simulink model "SF011A_EotLrng"  (R2013b)
settings: Solver=FixedStepDiscrete  SolverMode=SingleTasking  StartTime=0.0  StopTime=1  FixedStep=0.002  RelTol=1e-3
values from neighbouring files (symbols this model uses):
  ARCHGLBPRM_FLOATZEROTHD_ULS_F32 = DataDict.Constant    [SF011A_EotLrng_DataDict.m]
  CNVTOMILLISEC_MILLISECPERCNT_F32 = DataDict.Constant    [SF011A_EotLrng_DataDict.m]
  CORRLNFLT_CNT_U08 = DataDict.Constant    [SF011A_EotLrng_DataDict.m]
  DEBSTEP_CNT_U16 = DataDict.Constant    [SF011A_EotLrng_DataDict.m]
  EOTLIMDETD_CNT_LOGL = DataDict.Constant    [SF011A_EotLrng_DataDict.m]
  EOTLIMNOTDETD_CNT_LOGL = DataDict.Constant    [SF011A_EotLrng_DataDict.m]
  EotLrngAuthyStrtLrn = DataDict.Calibration    [SF011A_EotLrng_DataDict.m]
  EotLrngEotLrnTmr = DataDict.Calibration    [SF011A_EotLrng_DataDict.m]
  EotLrngHwAgOverTrvlCnt = DataDict.Calibration    [SF011A_EotLrng_DataDict.m]
  EotLrngHwAgOverTrvlEntr = DataDict.Calibration    [SF011A_EotLrng_DataDict.m]
  EotLrngHwAgOverTrvlExit = DataDict.Calibration    [SF011A_EotLrng_DataDict.m]
  EotLrngHwTqEotLrn = DataDict.Calibration    [SF011A_EotLrng_DataDict.m]
  EotLrngMotVelEotLrn = DataDict.Calibration    [SF011A_EotLrng_DataDict.m]
  EotLrngRackTrvlMax = DataDict.Calibration    [SF011A_EotLrng_DataDict.m]
  EotLrngRackTrvlMin = DataDict.Calibration    [SF011A_EotLrng_DataDict.m]
  EotLrngRstAuthyMin = DataDict.Calibration    [SF011A_EotLrng_DataDict.m]
  EotProtnRackTrvlLimrEna = DataDict.ImprtdCal    [SF011A_EotLrng_DataDict.m]
  HwAgOverTrvl = DataDict.NTC    [SF011A_EotLrng_DataDict.m]
  HWAGOVERTRVLMAXCNT_CNT_U08 = DataDict.Constant    [SF011A_EotLrng_DataDict.m]
  NODEBSTEP_CNT_U16 = DataDict.Constant    [SF011A_EotLrng_DataDict.m]
  OUTOFRNGFLT_CNT_U08 = DataDict.Constant    [SF011A_EotLrng_DataDict.m]
  RackEotStorgFlt = DataDict.NTC    [SF011A_EotLrng_DataDict.m]
  SIGAVLFLT_CNT_U08 = DataDict.Constant    [SF011A_EotLrng_DataDict.m]
undefined symbols (not defined in the file or in its folder): NtcSts1, NvmGetErrSts1, SigQlfr1
libraries: simulink x19, NxtrNvM x12, NxtrAbslt x5, NxtrLim x4, NxtrMax x3, NxtrMin x3
(part 4 of 7)

== system SF011A_EotLrng/EotLrng/EotLrngPer1/SRLNotEna/CalcResetEot ==
  HwAgDiDiagSts : Inport  RequirementInfo="{'linktype_rmi_doors' '0000ba59 (/E-STEER Core/SubSystem Specifications/Application Functions/SF011A Learned EOT Limits)' '#SF011A_79' 'true' 'REQ:  SF011A_79' '' } %GIDa_e08988e2_1562_4c51_b269_de6339d57bf1"
  HwAuthy : Inport  RequirementInfo="{'linktype_rmi_doors' '0000ba59 (/E-STEER Core/SubSystem Specifications/Application Functions/SF011A Learned EOT Limits)' '#SF011A_80' 'true' 'REQ:  SF011A_80' '' ; 'linktype_rmi_doors' '0000ba59 (/E-STEER Core/SubSystem Specifications/Application Functions/SF011A Learned EOT Limits)' '#SF011A_81' 'true' 'REQ:  SF011A_81' '' } %GIDa_5c7a69a0_a64f_4965_bcc2_68fe0bcf48ea"  Port=2
  HwAg : Inport  Port=3
  Calibration : Constant  RequirementInfo="{'linktype_rmi_doors' '0000ba59 (/E-STEER Core/SubSystem Specifications/Application Functions/SF011A Learned EOT Limits)' '#SF011A_80' 'true' 'REQ:  SF011A_80' '' ; 'linktype_rmi_doors' '0000ba59 (/E-STEER Core/SubSystem Specifications/Application Functions/SF011A Learned EOT Limits)' '#SF011A_81' 'true' 'REQ:  SF011A_81' '' } %GIDa_1b637f2f_e852_4a1f_a59d_2b9db53c6dd7"  Value=EotLrngRstAuthyMin
  Constant3 : Constant  RequirementInfo="{'linktype_rmi_doors' '0000ba59 (/E-STEER Core/SubSystem Specifications/Application Functions/SF011A Learned EOT Limits)' '#SF011A_80' 'true' 'REQ:  SF011A_80' '' ; 'linktype_rmi_doors' '0000ba59 (/E-STEER Core/SubSystem Specifications/Application Functions/SF011A Learned EOT Limits)' '#SF011A_81' 'true' 'REQ:  SF011A_81' '' } %GIDa_fd907c25_ae57_48e9_8be4_a6bebbc957dd"  Value=EotLrngRackTrvlMax
  Constant4 : Constant  RequirementInfo="{'linktype_rmi_doors' '0000ba59 (/E-STEER Core/SubSystem Specifications/Application Functions/SF011A Learned EOT Limits)' '#SF011A_81' 'true' 'REQ:  SF011A_81' '' ; 'linktype_rmi_doors' '0000ba59 (/E-STEER Core/SubSystem Specifications/Application Functions/SF011A Learned EOT Limits)' '#SF011A_80' 'true' 'REQ:  SF011A_80' '' } %GIDa_3d9f2888_eef3_40f6_8ef6_142645e82430"  Value=EotLrngRackTrvlMax
  CopyRight2 : Subsystem  Description=|  mask(Copyright Information){none=on}
      | Copyright info block.                                               
      |                                                                     
      | Place copyright information at the top of every subsystem in design.
      mask prompts: none "No parameters"
      mask help: Place copyright information at the top of every subsystem in design.
      mask Display:
      | NxtrConf = 'Nexteer Confidential';
      | 
      | sys = bdroot; %handle for the current model ("system")
      | first = get_param(sys,'Created');
      | if(isempty(first))
      |     first = datestr(now,'yyyy');
      | else
      |     first = first(end-3:end);  %year is last four digits
      | end
      | 
      | last = get_param(sys,'LastModifiedDate');
      | if isempty(last)
      |     last = datestr(now,'yyyy');
      | else
      |     last = last(end-3:end);
      | end
      | 
      | if strcmp(first,last)
      |     fprintf('%s -- Copyright %s Nexteer',NxtrConf,first)
      | else
      |     fprintf('%s -- %s%s- %s Nexteer',NxtrConf,char(169),first,last)
      | end
  Data Store Read1 : DataStoreRead  RequirementInfo="{'linktype_rmi_doors' '0000ba59 (/E-STEER Core/SubSystem Specifications/Application Functions/SF011A Learned EOT Limits)' '#SF011A_78' 'true' 'REQ:  SF011A_78' '' } %GIDa_dc92841a_08af_4fc8_a8e8_ed04e745d80a"  DataStoreName=RstLimReq
  Logical Operator : Logic  RequirementInfo="{'linktype_rmi_doors' '0000ba59 (/E-STEER Core/SubSystem Specifications/Application Functions/SF011A Learned EOT Limits)' '#SF011A_78' 'true' 'REQ:  SF011A_78' '' ; 'linktype_rmi_doors' '0000ba59 (/E-STEER Core/SubSystem Specifications/Application Functions/SF011A Learned EOT Limits)' '#SF011A_79' 'true' 'REQ:  SF011A_79' '' ; 'linktype_rmi_doors' '0000ba59 (/E-STEER Core/SubSystem Specifications/Application Functions/SF011A Learned EOT Limits)' '#SF011A_80' 'true' 'REQ:  SF011A_80' '' ; 'linktype_rmi_doors' '0000ba59 (/E-STEER Core/SubSystem Specifications/Application Functions/SF011A Learned EOT Limits)' '#SF011A_81' 'true' 'REQ:  SF011A_81' '' } %GIDa_11ff6ad1_50e6_4918_a9aa_75679ebe76f8"  Operator=OR  Inputs=3  AllPortsSameDT=off  OutDataTypeStr=boolean
  Logical Operator1 : Logic  RequirementInfo="{'linktype_rmi_doors' '0000ba59 (/E-STEER Core/SubSystem Specifications/Application Functions/SF011A Learned EOT Limits)' '#SF011A_80' 'true' 'REQ:  SF011A_80' '' ; 'linktype_rmi_doors' '0000ba59 (/E-STEER Core/SubSystem Specifications/Application Functions/SF011A Learned EOT Limits)' '#SF011A_81' 'true' 'REQ:  SF011A_81' '' } %GIDa_2555febd_936c_40b2_9f9b_c08210222f29"  Operator=OR  AllPortsSameDT=off  OutDataTypeStr=boolean
  Logical Operator2 : Logic  RequirementInfo="{'linktype_rmi_doors' '0000ba59 (/E-STEER Core/SubSystem Specifications/Application Functions/SF011A Learned EOT Limits)' '#SF011A_80' 'true' 'REQ:  SF011A_80' '' ; 'linktype_rmi_doors' '0000ba59 (/E-STEER Core/SubSystem Specifications/Application Functions/SF011A Learned EOT Limits)' '#SF011A_81' 'true' 'REQ:  SF011A_81' '' } %GIDa_6e14db6e_5a83_4e69_9a75_17202af61501"  AllPortsSameDT=off  OutDataTypeStr=boolean
  Relational Operator : RelationalOperator  RequirementInfo="{'linktype_rmi_doors' '0000ba59 (/E-STEER Core/SubSystem Specifications/Application Functions/SF011A Learned EOT Limits)' '#SF011A_80' 'true' 'REQ:  SF011A_80' '' ; 'linktype_rmi_doors' '0000ba59 (/E-STEER Core/SubSystem Specifications/Application Functions/SF011A Learned EOT Limits)' '#SF011A_81' 'true' 'REQ:  SF011A_81' '' } %GIDa_a3ca0082_78b3_49a3_89f7_5ece7a959c8e"  OutDataTypeStr=boolean
  Relational Operator2 : RelationalOperator  RequirementInfo="{'linktype_rmi_doors' '0000ba59 (/E-STEER Core/SubSystem Specifications/Application Functions/SF011A Learned EOT Limits)' '#SF011A_80' 'true' 'REQ:  SF011A_80' '' ; 'linktype_rmi_doors' '0000ba59 (/E-STEER Core/SubSystem Specifications/Application Functions/SF011A Learned EOT Limits)' '#SF011A_81' 'true' 'REQ:  SF011A_81' '' } %GIDa_389cdd7e_2d79_4d3e_a6fc_d51a3a0d06bf"  Operator=>  OutDataTypeStr=boolean
  Relational Operator3 : RelationalOperator  RequirementInfo="{'linktype_rmi_doors' '0000ba59 (/E-STEER Core/SubSystem Specifications/Application Functions/SF011A Learned EOT Limits)' '#SF011A_81' 'true' 'REQ:  SF011A_81' '' ; 'linktype_rmi_doors' '0000ba59 (/E-STEER Core/SubSystem Specifications/Application Functions/SF011A Learned EOT Limits)' '#SF011A_80' 'true' 'REQ:  SF011A_80' '' } %GIDa_7abd7096_ec6f_448b_88cf_8cd7c03d0901"  Operator=<  OutDataTypeStr=boolean
  Unary Minus : UnaryMinus  RequirementInfo="{'linktype_rmi_doors' '0000ba59 (/E-STEER Core/SubSystem Specifications/Application Functions/SF011A Learned EOT Limits)' '#SF011A_81' 'true' 'REQ:  SF011A_81' '' ; 'linktype_rmi_doors' '0000ba59 (/E-STEER Core/SubSystem Specifications/Application Functions/SF011A Learned EOT Limits)' '#SF011A_80' 'true' 'REQ:  SF011A_80' '' } %GIDa_d6db76b3_3df1_4d39_8e0a_09f1875fa956"
  RstEot : Outport  RequirementInfo="{'linktype_rmi_doors' '0000ba59 (/E-STEER Core/SubSystem Specifications/Application Functions/SF011A Learned EOT Limits)' '#SF011A_77' 'true' 'REQ:  SF011A_77' '' } %GIDa_90b21cd4_2507_4f0d_b885_ff293ec349f9"
  wires:
  Calibration/1 -> Relational Operator/2
  Relational Operator/1 -> Logical Operator2/1
  Data Store Read1/1 -> Logical Operator/1
  HwAgDiDiagSts/1 -> Logical Operator/2
  Logical Operator2/1 -> Logical Operator/3
  HwAuthy/1 -> Relational Operator/1
  Logical Operator/1 -> RstEot/1
  HwAg/1 -> Relational Operator2/1, Relational Operator3/1
  Constant4/1 -> Unary Minus/1
  Unary Minus/1 -> Relational Operator3/2
  Relational Operator2/1 -> Logical Operator1/1
  Relational Operator3/1 -> Logical Operator1/2
  Constant3/1 -> Relational Operator2/2
  Logical Operator1/1 -> Logical Operator2/2

== system SF011A_EotLrng/EotLrng/EotLrngPer1/SRLNotEna/CopyRight2 ==

== system SF011A_EotLrng/EotLrng/EotLrngPer1/SRLNotEna/LrnEotLim ==
  HwAuthy : Inport
  HwAg : Inport  Port=2
  HwTq : Inport  Port=3
  MotVelCrf : Inport  Port=4
  Action Port : ActionPort  ActionType=else
  CopyRight2 : Subsystem  Description=|  mask(Copyright Information){none=on}
      | Copyright info block.                                               
      |                                                                     
      | Place copyright information at the top of every subsystem in design.
      mask prompts: none "No parameters"
      mask help: Place copyright information at the top of every subsystem in design.
      mask Display:
      | NxtrConf = 'Nexteer Confidential';
      | 
      | sys = bdroot; %handle for the current model ("system")
      | first = get_param(sys,'Created');
      | if(isempty(first))
      |     first = datestr(now,'yyyy');
      | else
      |     first = first(end-3:end);  %year is last four digits
      | end
      | 
      | last = get_param(sys,'LastModifiedDate');
      | if isempty(last)
      |     last = datestr(now,'yyyy');
      | else
      |     last = last(end-3:end);
      | end
      | 
      | if strcmp(first,last)
      |     fprintf('%s -- Copyright %s Nexteer',NxtrConf,first)
      | else
      |     fprintf('%s -- %s%s- %s Nexteer',NxtrConf,char(169),first,last)
      | end
  LrgnEotCmplSts : Subsystem
  LrngEotLim : Subsystem
  wires:
  HwAg/1 -> [HwAg]
  [HwAg] -> LrngEotLim/2(HwAg)
  [HwAuthy] -> LrngEotLim/1(HwAuthy)
  HwAuthy/1 -> [HwAuthy]
  HwTq/1 -> LrgnEotCmplSts/3(HwTq)
  MotVelCrf/1 -> LrgnEotCmplSts/4(MotVelCrf)
  [HwAuthy] -> LrgnEotCmplSts/1(HwAuthy)
  [HwAg] -> LrgnEotCmplSts/2(HwAg)

== system SF011A_EotLrng/EotLrng/EotLrngPer1/SRLNotEna/RstEot ==
  note: 'ResetLimitRequest' is applicable only when SRL Enable is FALSE.
      | So 'IF' block is executed only when 'EotProtnRackTrvlLimrEna' is FALSE.
      |
      | Since ResetEot block is common across both 'Init' and 'Periodic',
      | 'EotProtnRackTrvlLimrEna' check is repeated here even though we know
      | 'EotProtnRackTrvlLimrEna' is FALSE inside this block.
      |
      | During Initalization, verifying 'EotProtnRackTrvlLimrEna' condition is appropriate as
      | NVM read and range check of EOT limits are common for both SRL enable and disable
      | conditions.
  Action Port : ActionPort  ActionType=then
  Cal1 : Constant  RequirementInfo="{'linktype_rmi_doors' '0000ba59 (/E-STEER Core/SubSystem Specifications/Application Functions/SF011A Learned EOT Limits)' '#SF011A_65' 'true' 'REQ:  SF011A_65' '' } %GIDa_d52bbe7c_f5dd_435b_a8ec_896b58cd087b"  Value=EotLrngRackTrvlMin
  Cal2 : Constant  RequirementInfo="{'linktype_rmi_doors' '0000ba59 (/E-STEER Core/SubSystem Specifications/Application Functions/SF011A Learned EOT Limits)' '#SF011A_66' 'true' 'REQ:  SF011A_66' '' } %GIDa_5c801997_1fa0_42fc_845b_823c2df2cccf"  Value=EotLrngRackTrvlMin
  Calibration4 : Constant  RequirementInfo={} %GIDa_95f2d169_28f3_4cc4_a9c4_9ddcc35cb0f1  Value=EotProtnRackTrvlLimrEna
  ChkRstLimReq : Subsystem  RequirementInfo="{'linktype_rmi_doors' '0000ba59 (/E-STEER Core/SubSystem Specifications/Application Functions/SF011A Learned EOT Limits)' '#SF011A_120' 'true' 'REQ:  SF011A_120' '' } %GIDa_0500a019_1cd4_48db_aadd_d6faf319209a"  TreatAsAtomicUnit=on
  Constant2 : Constant  RequirementInfo="{'linktype_rmi_doors' '0000ba59 (/E-STEER Core/SubSystem Specifications/Application Functions/SF011A Learned EOT Limits)' '#SF011A_67' 'true' 'REQ:  SF011A_67' '' } %GIDa_5cc54b8e_8cb3_405e_9244_9aa730592caf"  Value=EOTLIMNOTDETD_CNT_LOGL
  Constant3 : Constant  RequirementInfo="{'linktype_rmi_doors' '0000ba59 (/E-STEER Core/SubSystem Specifications/Application Functions/SF011A Learned EOT Limits)' '#SF011A_68' 'true' 'REQ:  SF011A_68' '' } %GIDa_f835e848_aaef_4e63_980b_8feb5e89ec22"  Value=EOTLIMNOTDETD_CNT_LOGL
  Copyright1 : Subsystem  Description=|  mask(Copyright Information){none=on}
      | Copyright info block.                                               
      |                                                                     
      | Place copyright information at the top of every subsystem in design.
      mask prompts: none "No parameters"
      mask help: Place copyright information at the top of every subsystem in design.
      mask Display:
      | NxtrConf = 'Nexteer Confidential';
      | 
      | sys = bdroot; %handle for the current model ("system")
      | first = get_param(sys,'Created');
      | if(isempty(first))
      |     first = datestr(now,'yyyy');
      | else
      |     first = first(end-3:end);  %year is last four digits
      | end
      | 
      | last = get_param(sys,'LastModifiedDate');
      | if isempty(last)
      |     last = datestr(now,'yyyy');
      | else
      |     last = last(end-3:end);
      | end
      | 
      | if strcmp(first,last)
      |     fprintf('%s\nCopyright  %s Nexteer',NxtrConf,first);
      | else
      |     fprintf('%s\n%s%s-%s Nexteer',NxtrConf,char(169),first,last);
      | end
  EotNotDetd : DataStoreWrite  RequirementInfo="{'linktype_rmi_doors' '0000ba59 (/E-STEER Core/SubSystem Specifications/Application Functions/SF011A Learned EOT Limits)' '#SF011A_65' 'true' 'REQ:  SF011A_65' '' ; 'linktype_rmi_doors' '0000ba59 (/E-STEER Core/SubSystem Specifications/Application Functions/SF011A Learned EOT Limits)' '#SF011A_66' 'true' 'REQ:  SF011A_66' '' ; 'linktype_rmi_doors' '0000ba59 (/E-STEER Core/SubSystem Specifications/Application Functions/SF011A Learned EOT Limits)' '#SF011A_67' 'true' 'REQ:  SF011A_67' '' ; 'linktype_rmi_doors' '0000ba59 (/E-STEER Core/SubSystem Specifications/Application Functions/SF011A Learned EOT Limits)' '#SF011A_68' 'true' 'REQ:  SF011A_68' '' } %GIDa_3262fe3b_a4e0_4e6e_9b27_5dd1eb6852a2"  DataStoreName=EotNvmData  DataStoreElements=EotNvmData.CwEot#EotNvmData.CcwEot#EotNvmData.CwEotDetd#EotNvmData.CcwEotDetd
  If1 : If  RequirementInfo={} %GIDa_d1d760e0_cfd7_4bc6_9717_51edf72193b9  IfExpression=~u1  ShowElse=off
  Unary Minus : UnaryMinus  RequirementInfo="{'linktype_rmi_doors' '0000ba59 (/E-STEER Core/SubSystem Specifications/Application Functions/SF011A Learned EOT Limits)' '#SF011A_66' 'true' 'REQ:  SF011A_66' '' } %GIDa_5788471f_d541_4b0b_bb6d_cefc2bdadbb3"
  wires:
  Cal1/1 -> EotNotDetd/1
  Constant2/1 -> EotNotDetd/3
  Constant3/1 -> EotNotDetd/4
  Cal2/1 -> Unary Minus/1
  Unary Minus/1 -> EotNotDetd/2
  Calibration4/1 -> If1/1
  If1/1 -> ChkRstLimReq/Action

== system SF011A_EotLrng/EotLrng/SerlComRstEot/SetRstLimReq/CopyRight2 ==

== system SF011A_EotLrng/EotLrng/EotLrngInit1/RstEot/ChkRstLimReq/CopyRight2 ==

== system SF011A_EotLrng/EotLrng/EotLrngInit1/RstEot/ChkRstLimReq/ResetLimReq ==
  Action Port : ActionPort  ActionType=then
  Constant : Constant  RequirementInfo="{'linktype_rmi_doors' '0000ba59 (/E-STEER Core/SubSystem Specifications/Application Functions/SF011A Learned EOT Limits)' '#SF011A_120' 'true' 'REQ:  SF011A_120' '' } %GIDa_f7b10d60_609c_4cee_b44d_5a3c1bacd354"  Value=false  OutDataTypeStr=boolean
  Copyright1 : Subsystem  Description=|  mask(Copyright Information){none=on}
      | Copyright info block.                                               
      |                                                                     
      | Place copyright information at the top of every subsystem in design.
      mask prompts: none "No parameters"
      mask help: Place copyright information at the top of every subsystem in design.
      mask Display:
      | NxtrConf = 'Nexteer Confidential';
      | 
      | sys = bdroot; %handle for the current model ("system")
      | first = get_param(sys,'Created');
      | if(isempty(first))
      |     first = datestr(now,'yyyy');
      | else
      |     first = first(end-3:end);  %year is last four digits
      | end
      | 
      | last = get_param(sys,'LastModifiedDate');
      | if isempty(last)
      |     last = datestr(now,'yyyy');
      | else
      |     last = last(end-3:end);
      | end
      | 
      | if strcmp(first,last)
      |     fprintf('%s\nCopyright  %s Nexteer',NxtrConf,first);
      | else
      |     fprintf('%s\n%s%s-%s Nexteer',NxtrConf,char(169),first,last);
      | end
  Update PIM3 : DataStoreWrite  RequirementInfo="{'linktype_rmi_doors' '0000ba59 (/E-STEER Core/SubSystem Specifications/Application Functions/SF011A Learned EOT Limits)' '#SF011A_120' 'true' 'REQ:  SF011A_120' '' } %GIDa_7eb83ca1_b4cc_406e_b3fa_ddc6c61849ca"  DataStoreName=RstLimReq
  wires:
  Constant/1 -> Update PIM3/1

== system SF011A_EotLrng/EotLrng/EotLrngInit1/SRLNotEna/GetRefTmr100MicroSec32bit/CopyRight2 ==

== system SF011A_EotLrng/EotLrng/EotLrngInit1/SetOverTrvlDiagcPass/SetNtcSts/CopyRight2 ==

== system SF011A_EotLrng/EotLrng/EotLrngPer1/HwAgCwAndCcwMax/HwAgCwAndCcw/CopyRight2 ==

== system SF011A_EotLrng/EotLrng/EotLrngPer1/HwAgCwAndCcwMax/HwAgCwAndCcw/MaxHwAgCcwDetd ==
  HwAg : Inport  RequirementInfo="{'linktype_rmi_doors' '0000ba59 (/E-STEER Core/SubSystem Specifications/Application Functions/SF011A Learned EOT Limits)' '#SF011A_156' 'true' 'REQ:  SF011A_156' '' } %GIDa_22f01cca_a8a8_4641_8e71_2cb13275130e"
  Action Port : ActionPort  ActionType=then
  CopyRight2 : Subsystem  Description=|  mask(Copyright Information){none=on}
      | Copyright info block.                                               
      |                                                                     
      | Place copyright information at the top of every subsystem in design.
      mask prompts: none "No parameters"
      mask help: Place copyright information at the top of every subsystem in design.
      mask Display:
      | NxtrConf = 'Nexteer Confidential';
      | 
      | sys = bdroot; %handle for the current model ("system")
      | first = get_param(sys,'Created');
      | if(isempty(first))
      |     first = datestr(now,'yyyy');
      | else
      |     first = first(end-3:end);  %year is last four digits
      | end
      | 
      | last = get_param(sys,'LastModifiedDate');
      | if isempty(last)
      |     last = datestr(now,'yyyy');
      | else
      |     last = last(end-3:end);
      | end
      | 
      | if strcmp(first,last)
      |     fprintf('%s -- Copyright %s Nexteer',NxtrConf,first)
      | else
      |     fprintf('%s -- %s%s- %s Nexteer',NxtrConf,char(169),first,last)
      | end
  MaxHwAgCcw : DataStoreWrite  RequirementInfo="{'linktype_rmi_doors' '0000ba59 (/E-STEER Core/SubSystem Specifications/Application Functions/SF011A Learned EOT Limits)' '#SF011A_156' 'true' 'REQ:  SF011A_156' '' } %GIDa_4af36dd2_28b5_4129_9beb_3e56c365343d"  DataStoreName=MaxHwAgCwAndCcw  DataStoreElements=MaxHwAgCwAndCcw.HwAgCcwMax
  Set Ram Block Status : NxtrNvM/Set Ram Block Status  RequirementInfo="{'linktype_rmi_doors' '0000ba59 (/E-STEER Core/SubSystem Specifications/Application Functions/SF011A Learned EOT Limits)' '#SF011A_156' 'true' 'REQ:  SF011A_156' '' } %GIDa_7c593be2_4683_4b3e_ada9_d0efb444baca"  FuncName=Set Ram Block Status  NvMBlockName=MaxHwAgCwAndCcw  VoidFuncRtn=on  BlockChanged_DSN=NvMSRBS_BlockChanged7  Return_DSN=NvMSRBS_Return7
      settings: AttributesFormatString=%<FuncName>
  WriteFlag : Constant  RequirementInfo="{'linktype_rmi_doors' '0000ba59 (/E-STEER Core/SubSystem Specifications/Application Functions/SF011A Learned EOT Limits)' '#SF011A_156' 'true' 'REQ:  SF011A_156' '' } %GIDa_329aef7b_d247_47c2_9367_373effa2ea02"  Value=true  OutDataTypeStr=boolean
      settings: AttributesFormatString=%<OutDataTypeStr>
  wires:
  HwAg/1 -> MaxHwAgCcw/1
  WriteFlag/1 -> Set Ram Block Status/1

== system SF011A_EotLrng/EotLrng/EotLrngPer1/HwAgCwAndCcwMax/HwAgCwAndCcw/MaxHwAgCwDetd ==
  HwAg : Inport  RequirementInfo="{'linktype_rmi_doors' '0000ba59 (/E-STEER Core/SubSystem Specifications/Application Functions/SF011A Learned EOT Limits)' '#SF011A_158' 'true' 'REQ:  SF011A_158' '' } %GIDa_3423f927_5b1e_412a_8572_0cfbd9588a53"
  Action Port : ActionPort  ActionType=then
  CopyRight2 : Subsystem  Description=|  mask(Copyright Information){none=on}
      | Copyright info block.                                               
      |                                                                     
      | Place copyright information at the top of every subsystem in design.
      mask prompts: none "No parameters"
      mask help: Place copyright information at the top of every subsystem in design.
      mask Display:
      | NxtrConf = 'Nexteer Confidential';
      | 
      | sys = bdroot; %handle for the current model ("system")
      | first = get_param(sys,'Created');
      | if(isempty(first))
      |     first = datestr(now,'yyyy');
      | else
      |     first = first(end-3:end);  %year is last four digits
      | end
      | 
      | last = get_param(sys,'LastModifiedDate');
      | if isempty(last)
      |     last = datestr(now,'yyyy');
      | else
      |     last = last(end-3:end);
      | end
      | 
      | if strcmp(first,last)
      |     fprintf('%s -- Copyright %s Nexteer',NxtrConf,first)
      | else
      |     fprintf('%s -- %s%s- %s Nexteer',NxtrConf,char(169),first,last)
      | end
  HwAgCwMax : DataStoreWrite  RequirementInfo="{'linktype_rmi_doors' '0000ba59 (/E-STEER Core/SubSystem Specifications/Application Functions/SF011A Learned EOT Limits)' '#SF011A_158' 'true' 'REQ:  SF011A_158' '' } %GIDa_ca6097d3_fcb9_4ceb_8c60_5655348f5a03"  DataStoreName=MaxHwAgCwAndCcw  DataStoreElements=MaxHwAgCwAndCcw.HwAgCwMax
  Set Ram Block Status : NxtrNvM/Set Ram Block Status  RequirementInfo="{'linktype_rmi_doors' '0000ba59 (/E-STEER Core/SubSystem Specifications/Application Functions/SF011A Learned EOT Limits)' '#SF011A_158' 'true' 'REQ:  SF011A_158' '' } %GIDa_0377f7b4_cb3b_443c_acbd_7b3854d0bb26"  FuncName=Set Ram Block Status  NvMBlockName=MaxHwAgCwAndCcw  VoidFuncRtn=on  BlockChanged_DSN=NvMSRBS_BlockChanged8  Return_DSN=NvMSRBS_Return8
      settings: AttributesFormatString=%<FuncName>
  WriteFlag : Constant  RequirementInfo="{'linktype_rmi_doors' '0000ba59 (/E-STEER Core/SubSystem Specifications/Application Functions/SF011A Learned EOT Limits)' '#SF011A_158' 'true' 'REQ:  SF011A_158' '' } %GIDa_9a95497a_03e5_4588_a188_3244d476b7ed"  Value=true  OutDataTypeStr=boolean
      settings: AttributesFormatString=%<OutDataTypeStr>
  wires:
  HwAg/1 -> HwAgCwMax/1
  WriteFlag/1 -> Set Ram Block Status/1

== system SF011A_EotLrng/EotLrng/EotLrngPer1/HwAgCwAndCcwMax/HwAgCwAndCcw/OverTrvlDiagc ==
  HwAg : Inport  RequirementInfo={} %GIDa_4bf3d064_8fb5_4b8f_8ab1_7ebbef85369d
  Action Port : ActionPort  ActionType=then
  " " : DataStoreRead  RequirementInfo="{'linktype_rmi_doors' '0000ba59 (/E-STEER Core/SubSystem Specifications/Application Functions/SF011A Learned EOT Limits)' '#SF011A_182' 'true' 'REQ:  SF011A_182' '' } %GIDa_5a4d0705_7441_4b8a_a391_a87d4a72cd43"  DataStoreName=HwAgOverTrvlCntrDi
  Abslt_f32_f32 : NxtrAbslt/Abslt_f32_f32  RequirementInfo="{'linktype_rmi_doors' '0000ba59 (/E-STEER Core/SubSystem Specifications/Application Functions/SF011A Learned EOT Limits)' '#SF011A_176' 'true' 'REQ:  SF011A_176' '' ; 'linktype_rmi_doors' '0000ba59 (/E-STEER Core/SubSystem Specifications/Application Functions/SF011A Learned EOT Limits)' '#SF011A_182' 'true' 'REQ:  SF011A_182' '' } %GIDa_0ac76e70_1def_40ef_a65a_8325cefdc2e3"  SFunctionSpec=single y1 = Abslt_f32_f32(single u1)
      settings: AttributesFormatString=%<Name>
  CntOvrTrvlAndSetNTC : Subsystem  RequirementInfo="{'linktype_rmi_doors' '0000ba59 (/E-STEER Core/SubSystem Specifications/Application Functions/SF011A Learned EOT Limits)' '#SF011A_208' 'true' 'REQ:  SF011A_208' '' ; 'linktype_rmi_doors' '0000ba59 (/E-STEER Core/SubSystem Specifications/Application Functions/SF011A Learned EOT Limits)' '#SF011A_176' 'true' 'REQ:  SF011A_176' '' } %GIDa_88b0f410_3b88_485f_8f70_fa4be7b1a518"  TreatAsAtomicUnit=on
  CopyRight2 : Subsystem  Description=|  mask(Copyright Information){none=on}
      | Copyright info block.                                               
      |                                                                     
      | Place copyright information at the top of every subsystem in design.
      mask prompts: none "No parameters"
      mask help: Place copyright information at the top of every subsystem in design.
      mask Display:
      | NxtrConf = 'Nexteer Confidential';
      | 
      | sys = bdroot; %handle for the current model ("system")
      | first = get_param(sys,'Created');
      | if(isempty(first))
      |     first = datestr(now,'yyyy');
      | else
      |     first = first(end-3:end);  %year is last four digits
      | end
      | 
      | last = get_param(sys,'LastModifiedDate');
      | if isempty(last)
      |     last = datestr(now,'yyyy');
      | else
      |     last = last(end-3:end);
      | end
      | 
      | if strcmp(first,last)
      |     fprintf('%s -- Copyright %s Nexteer',NxtrConf,first)
      | else
      |     fprintf('%s -- %s%s- %s Nexteer',NxtrConf,char(169),first,last)
      | end
  Data Store Write1 : DataStoreWrite  RequirementInfo="{'linktype_rmi_doors' '0000ba59 (/E-STEER Core/SubSystem Specifications/Application Functions/SF011A Learned EOT Limits)' '#SF011A_182' 'true' 'REQ:  SF011A_182' '' } %GIDa_31aa4f70_b05f_4d6d_8d41_742fe6df4d5a"  DataStoreName=HwAgOverTrvlCntrDi
  HwAgEntrCdn : Subsystem  RequirementInfo="{'linktype_rmi_doors' '0000ba59 (/E-STEER Core/SubSystem Specifications/Application Functions/SF011A Learned EOT Limits)' '#SF011A_176' 'true' 'REQ:  SF011A_176' '' } %GIDa_9f8f0f8a_dd9d_4310_821c_b1c366725007"
  HwAgExitCdn : Subsystem  RequirementInfo="{'linktype_rmi_doors' '0000ba59 (/E-STEER Core/SubSystem Specifications/Application Functions/SF011A Learned EOT Limits)' '#SF011A_182' 'true' 'REQ:  SF011A_182' '' } %GIDa_6943d643_83fd_4323_aebf_f83712e7efe1"
  If : If  RequirementInfo="{'linktype_rmi_doors' '0000ba59 (/E-STEER Core/SubSystem Specifications/Application Functions/SF011A Learned EOT Limits)' '#SF011A_176' 'true' 'REQ:  SF011A_176' '' ; 'linktype_rmi_doors' '0000ba59 (/E-STEER Core/SubSystem Specifications/Application Functions/SF011A Learned EOT Limits)' '#SF011A_182' 'true' 'REQ:  SF011A_182' '' ; 'linktype_rmi_doors' '0000ba59 (/E-STEER Core/SubSystem Specifications/Application Functions/SF011A Learned EOT Limits)' '#SF011A_211' 'true' 'REQ:  SF011A_211' '' } %GIDa_1134efe8_65e2_4184_b3f5_4cf2a495f9d9"  NumInputs=3  IfExpression=u1 & ~u3  ElseIfExpressions=u2 & u3
  Merge : Merge  RequirementInfo="{'linktype_rmi_doors' '0000ba59 (/E-STEER Core/SubSystem Specifications/Application Functions/SF011A Learned EOT Limits)' '#SF011A_182' 'true' 'REQ:  SF011A_182' '' } %GIDa_fa146c73_36e3_4ea4_994c_900d7b36f488"  Inputs=3
  Pass : Subsystem  RequirementInfo="{'linktype_rmi_doors' '0000ba59 (/E-STEER Core/SubSystem Specifications/Application Functions/SF011A Learned EOT Limits)' '#SF011A_182' 'true' 'REQ:  SF011A_182' '' ; 'linktype_rmi_doors' '0000ba59 (/E-STEER Core/SubSystem Specifications/Application Functions/SF011A Learned EOT Limits)' '#SF011A_176' 'true' 'REQ:  SF011A_176' '' } %GIDa_b1f841d4_4482_4d7c_83e6_0a4d7c5e708f"  TreatAsAtomicUnit=on
  RstHwAgOverTrvlSwtVari : Subsystem  RequirementInfo="{'linktype_rmi_doors' '0000ba59 (/E-STEER Core/SubSystem Specifications/Application Functions/SF011A Learned EOT Limits)' '#SF011A_182' 'true' 'REQ:  SF011A_182' '' } %GIDa_9742fada_1abe_4f6b_9351_51639d0766ac"  TreatAsAtomicUnit=on
  wires:
  HwAgEntrCdn/1(Out) -> If/1
  If/1 -> CntOvrTrvlAndSetNTC/Action
  HwAgExitCdn/1(Out) -> If/2
  If/2 -> RstHwAgOverTrvlSwtVari/Action
  If/3 -> Pass/Action
  " "/1 -> If/3
  CntOvrTrvlAndSetNTC/1(Out) -> Merge/1
  RstHwAgOverTrvlSwtVari/1(Out) -> Merge/2
  Pass/1(Out) -> Merge/3
  Merge/1 -> Data Store Write1/1
  HwAg/1 -> Abslt_f32_f32/1
  Abslt_f32_f32/1 -> HwAgExitCdn/1(HwAg), HwAgEntrCdn/1(HwAg)

== system SF011A_EotLrng/EotLrng/EotLrngPer1/SRLEna/ChkEotSigForNtc/CopyRight2 ==

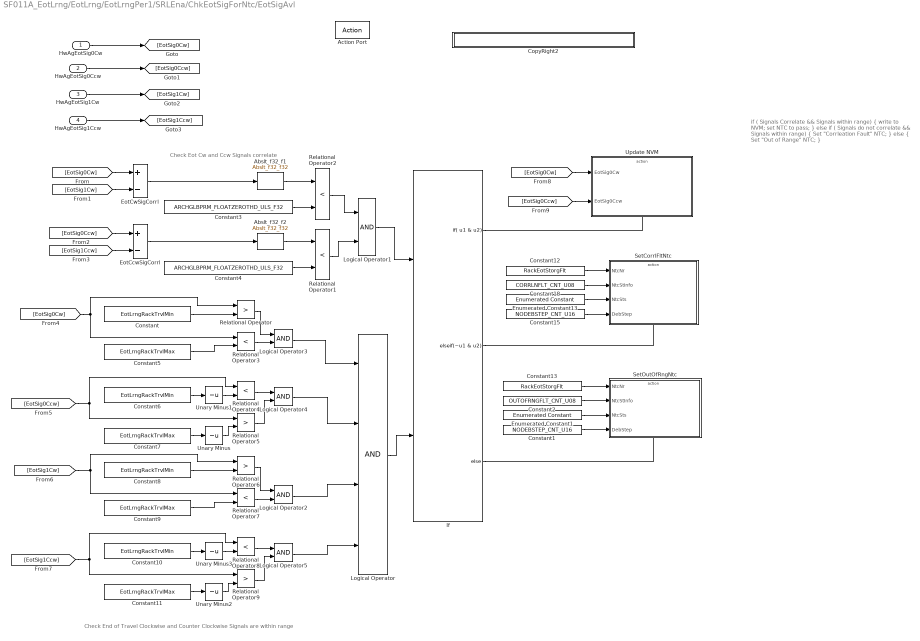
== system SF011A_EotLrng/EotLrng/EotLrngPer1/SRLEna/ChkEotSigForNtc/EotSigAvl ==
  note: if ( Signals Correlate && Signals within range)
      | {
      | 	 write to NVM;
      |   	 set NTC to pass;
      |  }
      | else if ( Signals do not correlate && Signals within range)
      | {
      | 	Set "Corrleation Fault" NTC;
      | }
      | else
      | {
      | 	Set "Out of Range" NTC;
      | }
  note: Check Eot Cw and Ccw Signals correlate
  note: Check End of Travel Clockwise and Counter Clockwise Signals are within range
  HwAgEotSig0Cw : Inport
  HwAgEotSig0Ccw : Inport  Port=2
  HwAgEotSig1Cw : Inport  Port=3
  HwAgEotSig1Ccw : Inport  Port=4
  Action Port : ActionPort  ActionType=then
  Abslt_f32_f1 : NxtrAbslt/Abslt_f32_f32  RequirementInfo="{'linktype_rmi_doors' '0000ba59 (/E-STEER Core/SubSystem Specifications/Application Functions/SF011A Learned EOT Limits)' '#SF011A_145' 'true' 'REQ:  SF011A_145' '' } %GIDa_dcbf7d67_a203_4a7b_acc1_c3c573cd02a8"  SFunctionSpec=single y1 = Abslt_f32_f32(single u1)
      settings: AttributesFormatString=%<Name>
  Abslt_f32_f2 : NxtrAbslt/Abslt_f32_f32  RequirementInfo="{'linktype_rmi_doors' '0000ba59 (/E-STEER Core/SubSystem Specifications/Application Functions/SF011A Learned EOT Limits)' '#SF011A_145' 'true' 'REQ:  SF011A_145' '' } %GIDa_9039b988_c4e9_48a7_8468_6a91edef9e93"  SFunctionSpec=single y1 = Abslt_f32_f32(single u1)
      settings: AttributesFormatString=%<Name>
  Constant : Constant  RequirementInfo="{'linktype_rmi_doors' '0000ba59 (/E-STEER Core/SubSystem Specifications/Application Functions/SF011A Learned EOT Limits)' '#SF011A_145' 'true' 'REQ:  SF011A_145' '' } %GIDa_377189a0_c038_468f_b453_e6e163f5020d"  Value=EotLrngRackTrvlMin
  Constant1 : Constant  RequirementInfo={} %GIDa_6e9739c0_027f_4f0e_97e0_b4b79b481585  Value=NODEBSTEP_CNT_U16
  Constant10 : Constant  RequirementInfo="{'linktype_rmi_doors' '0000ba59 (/E-STEER Core/SubSystem Specifications/Application Functions/SF011A Learned EOT Limits)' '#SF011A_145' 'true' 'REQ:  SF011A_145' '' } %GIDa_94c34584_70e8_4f1d_8de3_fe44f7ce5cc2"  Value=EotLrngRackTrvlMin
  Constant11 : Constant  RequirementInfo="{'linktype_rmi_doors' '0000ba59 (/E-STEER Core/SubSystem Specifications/Application Functions/SF011A Learned EOT Limits)' '#SF011A_145' 'true' 'REQ:  SF011A_145' '' } %GIDa_cbd55fcc_6658_4a9d_b17d_c159e8b9f8f8"  Value=EotLrngRackTrvlMax
  Constant12 : Constant  RequirementInfo={} %GIDa_0ef687e7_f9e2_4cd8_aeed_de3dbe45e309  Value=RackEotStorgFlt
  Constant13 : Constant  RequirementInfo={} %GIDa_a3e4fc3f_28b3_4291_8aec_e5827c4f21a3  Value=RackEotStorgFlt
  Constant15 : Constant  RequirementInfo={} %GIDa_d2736281_9e80_4023_ae62_1b64d6b7feda  Value=NODEBSTEP_CNT_U16
  Constant18 : Constant  RequirementInfo={} %GIDa_1395c2ec_9ae1_4e82_98d1_d104aa05a737  Value=CORRLNFLT_CNT_U08
  Constant2 : Constant  RequirementInfo={} %GIDa_4a2af044_cb51_45a8_9d47_77609114b212  Value=OUTOFRNGFLT_CNT_U08
  Constant3 : Constant  RequirementInfo="{'linktype_rmi_doors' '0000ba59 (/E-STEER Core/SubSystem Specifications/Application Functions/SF011A Learned EOT Limits)' '#SF011A_145' 'true' 'REQ:  SF011A_145' '' } %GIDa_f3de522e_f93a_4b41_8a64_b54f14745c7c"  Value=ARCHGLBPRM_FLOATZEROTHD_ULS_F32
  Constant4 : Constant  RequirementInfo="{'linktype_rmi_doors' '0000ba59 (/E-STEER Core/SubSystem Specifications/Application Functions/SF011A Learned EOT Limits)' '#SF011A_145' 'true' 'REQ:  SF011A_145' '' } %GIDa_c00bf581_9b75_4778_9195_63307b75df43"  Value=ARCHGLBPRM_FLOATZEROTHD_ULS_F32
  Constant5 : Constant  RequirementInfo="{'linktype_rmi_doors' '0000ba59 (/E-STEER Core/SubSystem Specifications/Application Functions/SF011A Learned EOT Limits)' '#SF011A_145' 'true' 'REQ:  SF011A_145' '' } %GIDa_52130ef0_d8a0_4af3_b16b_1c79bd2f5bc3"  Value=EotLrngRackTrvlMax
  Constant6 : Constant  RequirementInfo="{'linktype_rmi_doors' '0000ba59 (/E-STEER Core/SubSystem Specifications/Application Functions/SF011A Learned EOT Limits)' '#SF011A_145' 'true' 'REQ:  SF011A_145' '' } %GIDa_439c969b_0383_4a69_89eb_0827d607ed4a"  Value=EotLrngRackTrvlMin
  Constant7 : Constant  RequirementInfo="{'linktype_rmi_doors' '0000ba59 (/E-STEER Core/SubSystem Specifications/Application Functions/SF011A Learned EOT Limits)' '#SF011A_145' 'true' 'REQ:  SF011A_145' '' } %GIDa_19744b9d_4d33_464e_9f0b_9159a1ddb4bb"  Value=EotLrngRackTrvlMax
  Constant8 : Constant  RequirementInfo="{'linktype_rmi_doors' '0000ba59 (/E-STEER Core/SubSystem Specifications/Application Functions/SF011A Learned EOT Limits)' '#SF011A_145' 'true' 'REQ:  SF011A_145' '' } %GIDa_ae50bc88_8430_443d_b444_68640295ee7f"  Value=EotLrngRackTrvlMin
  Constant9 : Constant  RequirementInfo="{'linktype_rmi_doors' '0000ba59 (/E-STEER Core/SubSystem Specifications/Application Functions/SF011A Learned EOT Limits)' '#SF011A_145' 'true' 'REQ:  SF011A_145' '' } %GIDa_1808da1c_16c2_41b5_a3df_afebed5a0f63"  Value=EotLrngRackTrvlMax
  CopyRight2 : Subsystem  Description=|  mask(Copyright Information){none=on}
      | Copyright info block.                                               
      |                                                                     
      | Place copyright information at the top of every subsystem in design.
      mask prompts: none "No parameters"
      mask help: Place copyright information at the top of every subsystem in design.
      mask Display:
      | NxtrConf = 'Nexteer Confidential';
      | 
      | sys = bdroot; %handle for the current model ("system")
      | first = get_param(sys,'Created');
      | if(isempty(first))
      |     first = datestr(now,'yyyy');
      | else
      |     first = first(end-3:end);  %year is last four digits
      | end
      | 
      | last = get_param(sys,'LastModifiedDate');
      | if isempty(last)
      |     last = datestr(now,'yyyy');
      | else
      |     last = last(end-3:end);
      | end
      | 
      | if strcmp(first,last)
      |     fprintf('%s -- Copyright %s Nexteer',NxtrConf,first)
      | else
      |     fprintf('%s -- %s%s- %s Nexteer',NxtrConf,char(169),first,last)
      | end
  Enumerated Constant1 : simulink/Sources/Enumerated Constant  RequirementInfo={} %GIDa_365f942d_6fd3_46d3_adaf_33100c928908  OutDataTypeStr=Enum: NtcSts1  Value=NtcSts1.NTCSTS_FAILD  SampleTime=inf
  Enumerated Constant13 : simulink/Sources/Enumerated Constant  RequirementInfo={} %GIDa_eaaad463_243d_4a73_96e0_79c7a2001dc4  OutDataTypeStr=Enum: NtcSts1  Value=NtcSts1.NTCSTS_FAILD  SampleTime=inf
  EotCcwSigCorrl : Sum  RequirementInfo="{'linktype_rmi_doors' '0000ba59 (/E-STEER Core/SubSystem Specifications/Application Functions/SF011A Learned EOT Limits)' '#SF011A_145' 'true' 'REQ:  SF011A_145' '' } %GIDa_792a0f02_cc9d_49b4_87ce_30725f295e19"  Inputs=+-
  EotCwSigCorrl : Sum  RequirementInfo="{'linktype_rmi_doors' '0000ba59 (/E-STEER Core/SubSystem Specifications/Application Functions/SF011A Learned EOT Limits)' '#SF011A_145' 'true' 'REQ:  SF011A_145' '' } %GIDa_cc5e7958_4cc8_47d9_9592_b05d53447364"  Inputs=+-
  If : If  RequirementInfo="{'linktype_rmi_doors' '0000ba59 (/E-STEER Core/SubSystem Specifications/Application Functions/SF011A Learned EOT Limits)' '#SF011A_145' 'true' 'REQ:  SF011A_145' '' } %GIDa_7482c97f_6369_42c7_a57b_45b1dd7ce669"  NumInputs=2  IfExpression=u1 & u2  ElseIfExpressions=~u1 & u2
  Logical Operator : Logic  RequirementInfo="{'linktype_rmi_doors' '0000ba59 (/E-STEER Core/SubSystem Specifications/Application Functions/SF011A Learned EOT Limits)' '#SF011A_145' 'true' 'REQ:  SF011A_145' '' } %GIDa_ef8ab5b0_81f4_42d2_80b0_51f838e47681"  Inputs=4  AllPortsSameDT=off  OutDataTypeStr=boolean
  Logical Operator1 : Logic  RequirementInfo="{'linktype_rmi_doors' '0000ba59 (/E-STEER Core/SubSystem Specifications/Application Functions/SF011A Learned EOT Limits)' '#SF011A_145' 'true' 'REQ:  SF011A_145' '' } %GIDa_733b37d6_3119_467a_b2f7_e24824ce4b31"  AllPortsSameDT=off  OutDataTypeStr=boolean
  Logical Operator2 : Logic  RequirementInfo="{'linktype_rmi_doors' '0000ba59 (/E-STEER Core/SubSystem Specifications/Application Functions/SF011A Learned EOT Limits)' '#SF011A_145' 'true' 'REQ:  SF011A_145' '' } %GIDa_3f603afc_e87e_4b7a_b3f2_761255542193"  AllPortsSameDT=off  OutDataTypeStr=boolean
  Logical Operator3 : Logic  RequirementInfo="{'linktype_rmi_doors' '0000ba59 (/E-STEER Core/SubSystem Specifications/Application Functions/SF011A Learned EOT Limits)' '#SF011A_145' 'true' 'REQ:  SF011A_145' '' } %GIDa_b9ab3b1f_471a_4938_b1f6_9a9782440d82"  AllPortsSameDT=off  OutDataTypeStr=boolean
  Logical Operator4 : Logic  RequirementInfo="{'linktype_rmi_doors' '0000ba59 (/E-STEER Core/SubSystem Specifications/Application Functions/SF011A Learned EOT Limits)' '#SF011A_145' 'true' 'REQ:  SF011A_145' '' } %GIDa_b54d7ccf_5980_477d_9ac5_ffbfbfd3ee20"  AllPortsSameDT=off  OutDataTypeStr=boolean
  Logical Operator5 : Logic  RequirementInfo="{'linktype_rmi_doors' '0000ba59 (/E-STEER Core/SubSystem Specifications/Application Functions/SF011A Learned EOT Limits)' '#SF011A_145' 'true' 'REQ:  SF011A_145' '' } %GIDa_d8cb796b_490c_4e7f_b046_45a454ccbc57"  AllPortsSameDT=off  OutDataTypeStr=boolean
  Relational Operator : RelationalOperator  RequirementInfo="{'linktype_rmi_doors' '0000ba59 (/E-STEER Core/SubSystem Specifications/Application Functions/SF011A Learned EOT Limits)' '#SF011A_145' 'true' 'REQ:  SF011A_145' '' } %GIDa_4edb49f5_56f4_4496_ae9c_55abe9c2c7c3"  Operator=>  OutDataTypeStr=boolean
  Relational Operator1 : RelationalOperator  RequirementInfo="{'linktype_rmi_doors' '0000ba59 (/E-STEER Core/SubSystem Specifications/Application Functions/SF011A Learned EOT Limits)' '#SF011A_145' 'true' 'REQ:  SF011A_145' '' } %GIDa_115ce9aa_444e_4abf_96cc_d3307825babe"  Operator=<  OutDataTypeStr=boolean
  Relational Operator2 : RelationalOperator  RequirementInfo="{'linktype_rmi_doors' '0000ba59 (/E-STEER Core/SubSystem Specifications/Application Functions/SF011A Learned EOT Limits)' '#SF011A_145' 'true' 'REQ:  SF011A_145' '' } %GIDa_359ff840_6603_4c24_b326_dd69a425cdfe"  Operator=<  OutDataTypeStr=boolean
  Relational Operator3 : RelationalOperator  RequirementInfo="{'linktype_rmi_doors' '0000ba59 (/E-STEER Core/SubSystem Specifications/Application Functions/SF011A Learned EOT Limits)' '#SF011A_145' 'true' 'REQ:  SF011A_145' '' } %GIDa_a95215f1_e3f3_4f65_a54b_44da346f85fc"  Operator=<  OutDataTypeStr=boolean
  Relational Operator4 : RelationalOperator  RequirementInfo="{'linktype_rmi_doors' '0000ba59 (/E-STEER Core/SubSystem Specifications/Application Functions/SF011A Learned EOT Limits)' '#SF011A_145' 'true' 'REQ:  SF011A_145' '' } %GIDa_cc00be66_be59_445c_8901_01ea0f797452"  Operator=<  OutDataTypeStr=boolean
  Relational Operator5 : RelationalOperator  RequirementInfo="{'linktype_rmi_doors' '0000ba59 (/E-STEER Core/SubSystem Specifications/Application Functions/SF011A Learned EOT Limits)' '#SF011A_145' 'true' 'REQ:  SF011A_145' '' } %GIDa_ec132478_9c0a_49e7_a0b3_aaefbf24037f"  Operator=>  OutDataTypeStr=boolean
  Relational Operator6 : RelationalOperator  RequirementInfo="{'linktype_rmi_doors' '0000ba59 (/E-STEER Core/SubSystem Specifications/Application Functions/SF011A Learned EOT Limits)' '#SF011A_145' 'true' 'REQ:  SF011A_145' '' } %GIDa_6e24ce94_9708_49cb_98e3_e45f8c0adaaa"  Operator=>  OutDataTypeStr=boolean
  Relational Operator7 : RelationalOperator  RequirementInfo="{'linktype_rmi_doors' '0000ba59 (/E-STEER Core/SubSystem Specifications/Application Functions/SF011A Learned EOT Limits)' '#SF011A_145' 'true' 'REQ:  SF011A_145' '' } %GIDa_dae5cdc6_82d3_4d92_8285_b77459640b1f"  Operator=<  OutDataTypeStr=boolean
  Relational Operator8 : RelationalOperator  RequirementInfo="{'linktype_rmi_doors' '0000ba59 (/E-STEER Core/SubSystem Specifications/Application Functions/SF011A Learned EOT Limits)' '#SF011A_145' 'true' 'REQ:  SF011A_145' '' } %GIDa_119ec417_24b5_4c6f_a843_ed81e0625334"  Operator=<  OutDataTypeStr=boolean
  Relational Operator9 : RelationalOperator  RequirementInfo="{'linktype_rmi_doors' '0000ba59 (/E-STEER Core/SubSystem Specifications/Application Functions/SF011A Learned EOT Limits)' '#SF011A_145' 'true' 'REQ:  SF011A_145' '' } %GIDa_e05ca303_a29a_426d_a066_20160f050c91"  Operator=>  OutDataTypeStr=boolean
  SetCorrlFltNtc : Subsystem  RequirementInfo="{'linktype_rmi_doors' '0000ba59 (/E-STEER Core/SubSystem Specifications/Application Functions/SF011A Learned EOT Limits)' '#SF011A_166' 'true' 'REQ:  SF011A_166' '' ; 'linktype_rmi_doors' '0000ba59 (/E-STEER Core/SubSystem Specifications/Application Functions/SF011A Learned EOT Limits)' '#SF011A_167' 'true' 'REQ:  SF011A_167' '' ; 'linktype_rmi_doors' '0000ba59 (/E-STEER Core/SubSystem Specifications/Application Functions/SF011A Learned EOT Limits)' '#SF011A_23' 'true' 'REQ:  SF011A_23' '' } %GIDa_58185d81_63f4_4dbc_bfc3_b0d5e40a28e4"  mask(SetNTC){}
      mask help: SetNTC library block
  SetOutOfRngNtc : Subsystem  RequirementInfo="{'linktype_rmi_doors' '0000ba59 (/E-STEER Core/SubSystem Specifications/Application Functions/SF011A Learned EOT Limits)' '#SF011A_166' 'true' 'REQ:  SF011A_166' '' ; 'linktype_rmi_doors' '0000ba59 (/E-STEER Core/SubSystem Specifications/Application Functions/SF011A Learned EOT Limits)' '#SF011A_167' 'true' 'REQ:  SF011A_167' '' ; 'linktype_rmi_doors' '0000ba59 (/E-STEER Core/SubSystem Specifications/Application Functions/SF011A Learned EOT Limits)' '#SF011A_23' 'true' 'REQ:  SF011A_23' '' } %GIDa_abc55514_043a_4366_98dc_c134711c6fe3"  mask(SetNTC){}
      mask help: SetNTC library block
  Unary Minus : UnaryMinus  RequirementInfo="{'linktype_rmi_doors' '0000ba59 (/E-STEER Core/SubSystem Specifications/Application Functions/SF011A Learned EOT Limits)' '#SF011A_145' 'true' 'REQ:  SF011A_145' '' } %GIDa_e7d87cf3_f812_474d_8e9f_de69cbb86392"
  Unary Minus1 : UnaryMinus  RequirementInfo="{'linktype_rmi_doors' '0000ba59 (/E-STEER Core/SubSystem Specifications/Application Functions/SF011A Learned EOT Limits)' '#SF011A_145' 'true' 'REQ:  SF011A_145' '' } %GIDa_c5e34b2a_d31f_45b0_91a0_758aa2145b21"
  Unary Minus2 : UnaryMinus  RequirementInfo="{'linktype_rmi_doors' '0000ba59 (/E-STEER Core/SubSystem Specifications/Application Functions/SF011A Learned EOT Limits)' '#SF011A_145' 'true' 'REQ:  SF011A_145' '' } %GIDa_981cc8a7_bd01_4bea_92a2_9549087ba183"
  Unary Minus3 : UnaryMinus  RequirementInfo="{'linktype_rmi_doors' '0000ba59 (/E-STEER Core/SubSystem Specifications/Application Functions/SF011A Learned EOT Limits)' '#SF011A_145' 'true' 'REQ:  SF011A_145' '' } %GIDa_e37cdef2_1cc8_4298_90f6_27e3a30c2dad"
  Update NVM : Subsystem  RequirementInfo="{'linktype_rmi_doors' '0000ba59 (/E-STEER Core/SubSystem Specifications/Application Functions/SF011A Learned EOT Limits)' '#SF011A_145' 'true' 'REQ:  SF011A_145' '' } %GIDa_2222c6b4_4065_4214_87da_e8d8f93d01a9"  TreatAsAtomicUnit=on
  wires:
  If/1 -> Update NVM/Action
  HwAgEotSig0Cw/1 -> [EotSig0Cw]
  HwAgEotSig0Ccw/1 -> [EotSig0Ccw]
  HwAgEotSig1Cw/1 -> [EotSig1Cw]
  HwAgEotSig1Ccw/1 -> [EotSig1Ccw]
  [EotSig0Cw] -> EotCwSigCorrl/1
  [EotSig1Cw] -> EotCwSigCorrl/2
  Logical Operator1/1 -> If/1
  Logical Operator/1 -> If/2
  If/2 -> SetCorrlFltNtc/Action
  If/3 -> SetOutOfRngNtc/Action
  [EotSig0Cw] -> Update NVM/1(EotSig0Cw)
  [EotSig0Ccw] -> Update NVM/2(EotSig0Ccw)
  Constant15/1 -> SetCorrlFltNtc/4(DebStep)
  Enumerated Constant13/1 -> SetCorrlFltNtc/3(NtcSts)
  Constant18/1 -> SetCorrlFltNtc/2(NtcStInfo)
  Constant12/1 -> SetCorrlFltNtc/1(NtcNr)
  Constant13/1 -> SetOutOfRngNtc/1(NtcNr)
  Enumerated Constant1/1 -> SetOutOfRngNtc/3(NtcSts)
  Constant1/1 -> SetOutOfRngNtc/4(DebStep)
  Constant2/1 -> SetOutOfRngNtc/2(NtcStInfo)
  Relational Operator2/1 -> Logical Operator1/1
  Abslt_f32_f1/1 -> Relational Operator2/1
  Constant3/1 -> Relational Operator2/2
  EotCwSigCorrl/1 -> Abslt_f32_f1/1
  [EotSig0Ccw] -> EotCcwSigCorrl/1
  [EotSig1Ccw] -> EotCcwSigCorrl/2
  Relational Operator1/1 -> Logical Operator1/2
  Abslt_f32_f2/1 -> Relational Operator1/1
  Constant4/1 -> Relational Operator1/2
  EotCcwSigCorrl/1 -> Abslt_f32_f2/1
  [EotSig0Cw] -> Relational Operator3/1, Relational Operator/1
  Constant/1 -> Relational Operator/2
  Constant5/1 -> Relational Operator3/2
  Relational Operator/1 -> Logical Operator3/1
  Relational Operator3/1 -> Logical Operator3/2
  Logical Operator3/1 -> Logical Operator/1
  [EotSig0Ccw] -> Relational Operator5/1, Relational Operator4/1
  Constant6/1 -> Unary Minus1/1
  Constant7/1 -> Unary Minus/1
  Unary Minus/1 -> Relational Operator5/2
  Unary Minus1/1 -> Relational Operator4/2
  Relational Operator4/1 -> Logical Operator4/1
  Relational Operator5/1 -> Logical Operator4/2
  Logical Operator4/1 -> Logical Operator/2
  [EotSig1Cw] -> Relational Operator6/1, Relational Operator7/1
  Constant8/1 -> Relational Operator6/2
  Constant9/1 -> Relational Operator7/2
  Relational Operator6/1 -> Logical Operator2/1
  Relational Operator7/1 -> Logical Operator2/2
  Logical Operator2/1 -> Logical Operator/3
  [EotSig1Ccw] -> Relational Operator8/1, Relational Operator9/1
  Constant10/1 -> Unary Minus3/1
  Constant11/1 -> Unary Minus2/1
  Unary Minus2/1 -> Relational Operator9/2
  Unary Minus3/1 -> Relational Operator8/2
  Relational Operator8/1 -> Logical Operator5/1
  Relational Operator9/1 -> Logical Operator5/2
  Logical Operator5/1 -> Logical Operator/4

== system SF011A_EotLrng/EotLrng/EotLrngPer1/SRLEna/ChkEotSigForNtc/SetSigAvlFltNtc ==
  NtcNr : Inport
  NtcStInfo : Inport  Port=2
  NtcSts : Inport  Port=3
  DebStep : Inport  Port=4
  CallDiagMgr : ActionPort  ActionType=else
  SetNtcSts : Subsystem  RequirementInfo={} %GIDa_f4fae4d2_d65b_41d3_94db_e8a6b16d88bb  TreatAsAtomicUnit=on
      settings: RTWSystemCode=Inline
  wires:
  NtcNr/1 -> SetNtcSts/1(NtcNr)  "NtcNr"
  NtcSts/1 -> SetNtcSts/3(NtcSts)
  DebStep/1 -> SetNtcSts/4(DebStep)
  NtcStInfo/1 -> SetNtcSts/2(NtcStInfo)

== system SF011A_EotLrng/EotLrng/EotLrngPer1/SRLEna/GetNtcQlfrSts/CopyRight2 ==

== system SF011A_EotLrng/EotLrng/EotLrngPer1/SRLNotEna/CalcResetEot/CopyRight2 ==

== system SF011A_EotLrng/EotLrng/EotLrngPer1/SRLNotEna/LrnEotLim/CopyRight2 ==
